simulink model "stm32f4_data_logger_ascii_rtc_demo"  (Simulink 7.3)
settings: Solver=FixedStepDiscrete  SolverMode=SingleTasking  StartTime=0.0  StopTime=10.0  RelTol=1e-3
PreLoadFcn:
  | waijung.modelPreload; % Required for working with Waijung Blockset. Do not remove.
undefined symbols (not defined in the file): HSEOSC, Link, LQFP176, ST, STM32F417IG
libraries: simulink x17, stm32f4_sdio_lib x1, stm32f4_io_lib x1, stm32f4_adc_lib x1, stm32f4_device_config_lib x1
CloseFcn:
  | waijung.modelClose; % Required for working with Waijung Blockset. Do not remove.
settings Model: Creator=Krisada  LastModifiedBy=Krisada
settings OptimizationCC: OptimizeModelRefInitCode=on  LifeSpan=1
settings HardwareCC: ProdEndianess=LittleEndian  ProdHWDeviceType=ARM Compatible->Cortex - M4  TargetEndianess=LittleEndian  TargetHWDeviceType=ARM Compatible->Cortex - M4
settings RTWCC: SystemTargetFile=stm32f4.tlc  GenerateMakefile=off  TemplateMakefile=ert_default_tmf  Description=STM32F4 Target  ProcessScript=stm32f4_make_rtw_hook
settings CodeAppCC: IgnoreCustomStorageClasses=off
settings STFCustomTargetCC: ModelReferenceCompliant=off  CombineOutputUpdateFcns=on  ERTCustomFileBanners=on  SupportContinuousTime=off  SupportNonInlinedSFcns=off  SystemTargetFile=stm32f4.tlc
settings ERTTargetCC: MultiwordLength=2048  ModelReferenceCompliant=off  ParMdlRefBuildCompliant=off  CompOptLevelCompliant=off  ERTFirstTimeCompliant=off  ModelStepFunctionPrototypeControlCompliant=off  CPPClassGenCompliant=off  ExtModeMexFile=noextcomm  InlinedParameterPlacement=NonHierarchical  ERTSrcFileBannerTemplate=stm32f4_code_template.cgt  ERTHdrFileBannerTemplate=stm32f4_code_template.cgt  ERTDataSrcFileTemplate=stm32f4_code_template.cgt  ERTDataHdrFileTemplate=stm32f4_code_template.cgt  ERTCustomFileTemplate=stm32f4_file_process.tlc

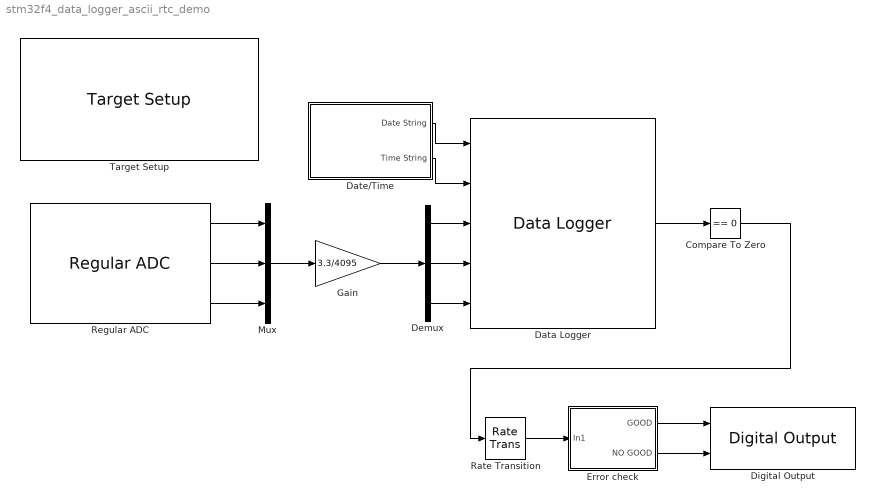
== system stm32f4_data_logger_ascii_rtc_demo ==
  Compare To Zero : simulink/Logic and Bit Operations/Compare To Zero  SystemSampleTime=-1  relop===  LogicOutDataTypeMode=uint8  ZeroCross=off
  Data Logger : stm32f4_sdio_lib/Data Logger  variablefilename=off  filename='data.csv'  conf=DataLogger  transfer=Blocking  packet=Ascii  header='Date,Time,data1,data2,data3\r\n'  asciiformat='%s,%s,%f,%f,%f,\r\n'  porttype_double=2  porttype_single=0  porttype_int8=0  porttype_uint8=1  porttype_int16=0  porttype_uint16=0  porttype_int32=0  porttype_uint32=0  advance=off  buffersize=2048  safeprintf=on  createfileoptions=Rename  synctimer=1  enablestatus=on  portpinstr=0  sampletime=-1  blockid=DataLogger  inputporttype=[-1,-1,-1,-1,-1]  inputportwidth=[1,1,1,1,1]  inputportlabel={'D0 (string)','D1 (string)','D2 (single)','D3 (single)','D4 (single)'}  outputporttype=[3]  outputportwidth=[1]  outputportlabel={'Status'}  compat=0  optionstring="[\"on\",\"off\",\"data.csv\",\"Ascii\",\"2048\",\"?\",\"?\",\"on\",\"1000000\",\"Rename\",\"-\",\"-\",\"-\",\"-\",\"-\",\"char *\",\"char *\",\"float\",\"float\",\"float\"]"
  Date/Time : Subsystem
  Demux : Demux  Outputs=3
  Digital Output : stm32f4_io_lib/Digital Output  use_bitband=on  port=D  speed=100  porttype=Push Pull  porttypestr=PP  use_pin0=off  use_pin1=off  use_pin2=off  use_pin3=off  use_pin4=off  use_pin5=off  use_pin6=off  use_pin7=off  use_pin8=off  use_pin9=off  use_pin10=off  use_pin11=off  use_pin12=on  use_pin13=on  use_pin14=off  use_pin15=off  pinstr=GPIO_Pin_12 | GPIO_Pin_13  usedpinarray="[0  0  0  0  0  0  0  0  0  0  0  0  1  1  0  0]"  bitbandingstr=|  sampletime=-1  sampletimestr=0.1  blockid=DigitalOutput  enablecustomportlabel=off  globalinit=off  cinputportlabel=In1, In2  coutputportlabel=0
      | #define DigitalOutput_D12 Peripheral_BB(GPIOD->ODR, 12)  /* Output pin */
      | #define DigitalOutput_D13 Peripheral_BB(GPIOD->ODR, 13)  /* Output pin */
  Error check : Subsystem
  Gain : Gain  Gain=3.3/4095  ParameterDataType=fixdt(1, 16)  ParameterScaling=2^0  OutDataType=fixdt(1, 16)  OutScaling=2^0  OutDataTypeStr=Inherit: Same as input  ParamDataTypeStr=Inherit: Same as input
  Mux : Mux  Inputs=3
  Rate Transition : RateTransition  OutPortSampleTime=0.1
  Regular ADC : stm32f4_adc_lib/Regular ADC  Priority=1  adcmodule=1  outputdatatype=Single  prescaler=2  prescalerstr=ADC_Prescaler_Div2  chsamplingtime=Auto  chsamplingtimestr=ADC_SampleTime_480Cycles  read_an0=off  read_an1=off  read_an2=off  read_an3=off  read_an4=off  read_an5=on  read_an6=on  read_an7=on  read_an8=off  read_an9=off  read_an10=off  read_an11=off  read_an12=off  read_an13=off  read_an14=off  read_an15=off  read_an16=off  read_an17=off  read_an18=off  pinstr=GPIO_Pin_5 | GPIO_Pin_6 | GPIO_Pin_7  usedpinarray="[0  0  0  0  0  1  1  1  0  0  0  0  0  0  0  0  0  0  0]"  usedportidarray="[0  0  0]"  usedpinidarray="[5  6  7]"  usedpinidcount=3  sampletime=0.5  blockid=RegularADC  enablecustomportlabel=off  cinputportlabel=0  coutputportlabel=Out1, Out2
  Target Setup : stm32f4_device_config_lib/Target Setup  Priority=100  compiler=GNU ARM  previous_compiler=GNU ARM  mcu=STM32F417IG (LQFP176)  mcustr=STM32F417IG  clockconfig=HSEOSC-8MHz  system_stm32f4xx_c_path=F:\trunk\targets\stm32f4_target\stm32f4\utils\system_stm32f4xx_default\STM32F40_41xxx\hseosc8mhz  showmemoryconfiguration=off  stacksize=0x2000  heapsize=0x2000  enableautocompiledownload=on  fullchiperase=off  programmerinterface=ST-Link  editctrlstr=on  compilercontrolstr=$(patsubst %, -I%, .) -mcpu=cortex-m4 -mthumb -mthumb-interwork -mfloat-abi=hard -mfpu=fpv4-sp-d16 -ffast-math -Wall -Wextra -Ofast  assemblercontrolstr=$(patsubst %, -I%, .) -mcpu=cortex-m4 -mthumb -mthumb-interwork -mfloat-abi=hard -mfpu=fpv4-sp-d16 -ffast-math -Wall -Wextra -Ofast -Wa,-amhls=$(<:.s=.lst) -D__STACK_SIZE=$(STACK_SIZE) -D__HEAP_SIZE=$(HEAP_SIZE)  linkercontrolstr=-T$(LD_SCRIPT) -g -Wl,-Map=$(MAP),--cref,--no-warn-mismatch -mcpu=cortex-m4 -mthumb -mthumb-interwork -mfloat-abi=hard -mfpu=fpv4-sp-d16 -specs=nosys.specs  runafterdownload=on  execprofile=None  profileruart=3  profilerbaud=500000  profilertxpin=D8  profilerinitstr=0.01,168000000,1680000,500000,0  manualsetsampletime=off  sampletime=0.01  blockid=TargetSetup  systickreloadvalue=1680000  hseval=8000000  lastprofileruart=3  hclk=168000000  flashorigin=0x8000000  flashlength=1024k  ramorigin=0x20000000  ramlength=128k  useextram=off
  wires:
  Data Logger/1 -> Compare To Zero/1
  Compare To Zero/1 -> Rate Transition/1
  Error check/1(GOOD) -> Digital Output/1
  Error check/2(NO GOOD) -> Digital Output/2
  Rate Transition/1 -> Error check/1(In1)
  Gain/1 -> Demux/1
  Mux/1 -> Gain/1
  Regular ADC/2 -> Mux/2
  Regular ADC/1 -> Mux/1
  Regular ADC/3 -> Mux/3
  Demux/3 -> Data Logger/5
  Demux/2 -> Data Logger/4
  Demux/1 -> Data Logger/3
  Date/Time/2(Time String) -> Data Logger/2
  Date/Time/1(Date String) -> Data Logger/1

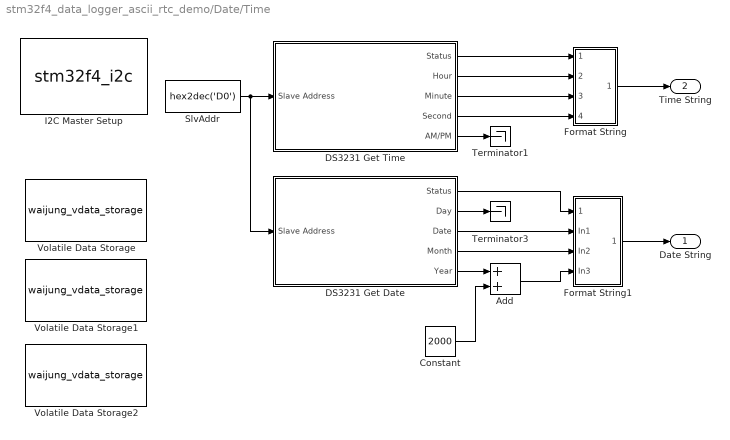
== system stm32f4_data_logger_ascii_rtc_demo/Date/Time ==
  Add : Sum  OutDataType=fixdt(1, 16)  OutScaling=2^-10
  Constant : Constant  Value=2000  OutDataTypeMode=uint32  OutDataType=fixdt(1, 16)  OutScaling=2^0  OutDataTypeStr=uint32
  DS3231 Get Date : Subsystem  mask{blockfunction=date, module=1}
      mask prompts: blockfunction "Function"; module "I2C module"
      mask init:
      | amg_high_precision_rtc_callback('init');
      mask Help: web(fullfile(waijungdocroot,'DS3231_Get_Date.htm'), '-browser')
      mask StyleString: popup(temp|time|date),popup(1|2|3)
      mask CallbackString: |amg_high_precision_rtc_callback('module');
      mask Display: text(0.5, 0.5, 'Port: I2C1','ver','middle','hor','center');port_label('input', 1,'SlvAddr');port_label('output', 1,'Status');port_label('output', 2,'Day(1-7)');port_label('output', 3,'Date(1-31)');port_label('output', 4,'Month(1-12)');port_label('output', 5,'Year(0-99)');
  DS3231 Get Time : Subsystem  mask{blockfunction=time, module=1}
      mask prompts: blockfunction "Function"; module "I2C module"
      mask init:
      | amg_high_precision_rtc_callback('init');
      mask Help: web(fullfile(waijungdocroot,'DS3231_Get_Time.htm'), '-browser')
      mask StyleString: popup(temp|time|date),popup(1|2|3)
      mask CallbackString: |amg_high_precision_rtc_callback('module');
      mask Display: text(0.5, 0.5, 'Port: I2C1','ver','middle','hor','center');port_label('input', 1,'SlvAddr');port_label('output', 1,'Status');port_label('output', 2,'Hour(0-11/23)');port_label('output', 3,'Minute(0-59)');port_label('output', 4,'Second(0-59)');port_label('output', 5,'AM(0)/PM(1)');
  Format String : Subsystem
  Format String1 : Subsystem
  I2C Master Setup : S-Function  FunctionName=stm32f4_i2c  Parameters=configuration,module,transfer,clkspeed,timeout,sdapin,sclpin,writecount,readcount,inputtypearray,outputtypearray,confstr,sampletime,sampletimestr,blockid  EnableBusSupport=off  mask(stm32f4_i2c){configuration=Setup, module=1, lastmodule=1, transfer=Blocking, dutycycle=TLow/THigh = 2, clkspeed=100, timeout=25, writecount=0, readcount=0, sdapin=B7, sclpin=B6, waitwritetime=0, inputtypearray=[0], outputtypearray=[0], confstr=["B","7","B","6","1","1","6","0","I2C_DutyCycle_2","0","off"], sampletime=-1, sampletimestr=0.01, blockid=DateTimeI2CMasterSetup}
      mask prompts: module "I2C Module"; lastmodule "Last module"; transfer "Transfer mode"; dutycycle "Duty cycle in fast mode"; clkspeed "Clock speed (kHz)"; timeout "Timeout (ms)"; writecount "Bytes write count"; readcount "Bytes read count"; sdapin "SDA pin"; sclpin "SCL pin"; waitwritetime "Wait write time (ms), default is 0"; inputtypearray "Input type array"; outputtypearray "Output type array"; confstr "Configuration string"; sampletime "Sample time (sec)"; sampletimestr "Compiled sample time (sec) in string"
      mask init:
      | stm32f4_i2c_callback('init');
      mask Help: web(fullfile(waijungdocroot,'stm32f4_i2c_setup.htm'), '-browser')
      mask StyleString: popup(Setup|Transaction),popup(1|2|3),edit,popup(Blocking|Non-blocking),popup(TLow/THigh = 16/9|TLow/THigh = 2),edit,edit,edit,edit,popup(Not used|B7|B9),popup(Not used|B6|B8),edit,edit,edit,edit,edit,edit,edit
      mask CallbackString: stm32f4_i2c_callback('configuration');|stm32f4_i2c_callback('module');|||stm32f4_i2c_callback('dutycycle');|||stm32f4_i2c_callback('writecount');|stm32f4_i2c_callback('readcount');|stm32f4_i2c_callback('sdapin');|stm32f4_i2c_callback('sclpin');||||stm32f4_i2c_callback('confstr');|stm32f4_i2c_callback('sampletime');|stm32f4_i2c_callback('sampletimestr');|stm32f4_i2c_callback('blockid');
      mask Display: text(0.5, 0.5, 'Module: I2C1\nClock: 100kHz\nSDA/SCL Pin: B7/B6','ver','middle','hor','center');
  SlvAddr : Constant  Priority=0  Value=hex2dec('D0')  OutDataTypeMode=uint8  OutDataType=fixdt(1, 16)  OutScaling=2^0  OutDataTypeStr=uint8
  Terminator1 : Terminator
  Terminator3 : Terminator
  Volatile Data Storage : S-Function  FunctionName=waijung_vdata_storage  Parameters=storagetype,storagename,initval,varname,buffersize,initvalstring,sampletime,sampletimestr,blockid,storagetypestr  EnableBusSupport=off  mask(waijung_vdata_storage){storagetype=string, storagename=date_str, initval=0, varname=DateTimeVolatileDataStorage_date_str, buffersize=64, initvalstring='', webintegration=Disable, weboutputformat='%s', webcgicallback=(void*)0, laststoragetype=string, sampletime=-1, sampletimestr=0.01, blockid=DateTimeVolatileDataStorage, storagetypestr=char}
      mask prompts: storagetype "Storage Type"; storagename "Storage Name (must be a valid variable name)"; initval "Initial value (Apply at Power on Reset only)"; varname "Variable name"; buffersize "Size (bytes)"; initvalstring "Initial value (Apply at Power on Reset only)"; webintegration "Web CGI varget/varset integration"; weboutputformat "Web CGI varget output format"; webcgicallback "Web CGI varset callback"; laststoragetype "Last selected Storage Type"; sampletime "Sample time (sec)"; sampletimestr "Compiled sample time (sec) in string"; storagetypestr "Type string"
      mask help:
      | This block implements a volatile Data Storage.
      |
      | Web CGI varset/varget integratiopn:
      | Enable - In webserver application, allow remote access via http.
      | Disable - Variable is use in local only.
      mask init:
      | waijung_vdata_storage_callback('init');
      mask Help: web(fullfile(waijungdocroot,'Volatile_Data_Storage.htm'))
      mask StyleString: popup(double|single|uint32|int32|uint16|int16|uint8|int8|string),edit,edit,edit,edit,edit,popup(Disable|ReadOnly|Write/ Read|ReadOnly with KeyValuePair|Write/ Read with KeyValuePair),edit,edit,popup(double|single|uint32|int32|uint16|int16|uint8|int8|string),edit,edit,edit,edit
      mask CallbackString: waijung_vdata_storage_callback('storagetype');|waijung_vdata_storage_callback('storagename');|waijung_vdata_storage_callback('initval');|waijung_vdata_storage_callback('varname');||waijung_vdata_storage_callback('initvalstring');|waijung_vdata_storage_callback('webintegration');|waijung_vdata_storage_callback('weboutputformat');|||waijung_vdata_storage_callback('sampletime');|waijung_vdata_storage_callback('sampletimestr');|waijung_vdata_storage_callback('blockid');|
      mask Display: text(0.5, 0.5, 'Name: date_str\nType: string','ver','middle','hor','center')
  Volatile Data Storage1 : S-Function  FunctionName=waijung_vdata_storage  Parameters=storagetype,storagename,initval,varname,buffersize,initvalstring,sampletime,sampletimestr,blockid,storagetypestr  EnableBusSupport=off  mask(waijung_vdata_storage){storagetype=string, storagename=time_str, initval=0, varname=DateTimeVolatileDataStorage1_time_str, buffersize=64, initvalstring='', webintegration=Disable, weboutputformat='%s', webcgicallback=(void*)0, laststoragetype=string, sampletime=-1, sampletimestr=0.01, blockid=DateTimeVolatileDataStorage1, storagetypestr=char}
      mask prompts: storagetype "Storage Type"; storagename "Storage Name (must be a valid variable name)"; initval "Initial value (Apply at Power on Reset only)"; varname "Variable name"; buffersize "Size (bytes)"; initvalstring "Initial value (Apply at Power on Reset only)"; webintegration "Web CGI varget/varset integration"; weboutputformat "Web CGI varget output format"; webcgicallback "Web CGI varset callback"; laststoragetype "Last selected Storage Type"; sampletime "Sample time (sec)"; sampletimestr "Compiled sample time (sec) in string"; storagetypestr "Type string"
      mask help:
      | This block implements a volatile Data Storage.
      |
      | Web CGI varset/varget integratiopn:
      | Enable - In webserver application, allow remote access via http.
      | Disable - Variable is use in local only.
      mask init:
      | waijung_vdata_storage_callback('init');
      mask Help: web(fullfile(waijungdocroot,'Volatile_Data_Storage.htm'))
      mask StyleString: popup(double|single|uint32|int32|uint16|int16|uint8|int8|string),edit,edit,edit,edit,edit,popup(Disable|ReadOnly|Write/ Read|ReadOnly with KeyValuePair|Write/ Read with KeyValuePair),edit,edit,popup(double|single|uint32|int32|uint16|int16|uint8|int8|string),edit,edit,edit,edit
      mask CallbackString: waijung_vdata_storage_callback('storagetype');|waijung_vdata_storage_callback('storagename');|waijung_vdata_storage_callback('initval');|waijung_vdata_storage_callback('varname');||waijung_vdata_storage_callback('initvalstring');|waijung_vdata_storage_callback('webintegration');|waijung_vdata_storage_callback('weboutputformat');|||waijung_vdata_storage_callback('sampletime');|waijung_vdata_storage_callback('sampletimestr');|waijung_vdata_storage_callback('blockid');|
      mask Display: text(0.5, 0.5, 'Name: time_str\nType: string','ver','middle','hor','center')
  Volatile Data Storage2 : S-Function  FunctionName=waijung_vdata_storage  Parameters=storagetype,storagename,initval,varname,buffersize,initvalstring,sampletime,sampletimestr,blockid,storagetypestr  EnableBusSupport=off  mask(waijung_vdata_storage){storagetype=string, storagename=date_time_error, initval=0, varname=DateTimeVolatileDataStorage2_date_time_error, buffersize=64, initvalstring='Error', webintegration=Disable, weboutputformat='%s', webcgicallback=(void*)0, laststoragetype=string, sampletime=-1, sampletimestr=0.01, blockid=DateTimeVolatileDataStorage2, storagetypestr=char}
      mask prompts: storagetype "Storage Type"; storagename "Storage Name (must be a valid variable name)"; initval "Initial value (Apply at Power on Reset only)"; varname "Variable name"; buffersize "Size (bytes)"; initvalstring "Initial value (Apply at Power on Reset only)"; webintegration "Web CGI varget/varset integration"; weboutputformat "Web CGI varget output format"; webcgicallback "Web CGI varset callback"; laststoragetype "Last selected Storage Type"; sampletime "Sample time (sec)"; sampletimestr "Compiled sample time (sec) in string"; storagetypestr "Type string"
      mask help:
      | This block implements a volatile Data Storage.
      |
      | Web CGI varset/varget integratiopn:
      | Enable - In webserver application, allow remote access via http.
      | Disable - Variable is use in local only.
      mask init:
      | waijung_vdata_storage_callback('init');
      mask Help: web(fullfile(waijungdocroot,'Volatile_Data_Storage.htm'))
      mask StyleString: popup(double|single|uint32|int32|uint16|int16|uint8|int8|string),edit,edit,edit,edit,edit,popup(Disable|ReadOnly|Write/ Read|ReadOnly with KeyValuePair|Write/ Read with KeyValuePair),edit,edit,popup(double|single|uint32|int32|uint16|int16|uint8|int8|string),edit,edit,edit,edit
      mask CallbackString: waijung_vdata_storage_callback('storagetype');|waijung_vdata_storage_callback('storagename');|waijung_vdata_storage_callback('initval');|waijung_vdata_storage_callback('varname');||waijung_vdata_storage_callback('initvalstring');|waijung_vdata_storage_callback('webintegration');|waijung_vdata_storage_callback('weboutputformat');|||waijung_vdata_storage_callback('sampletime');|waijung_vdata_storage_callback('sampletimestr');|waijung_vdata_storage_callback('blockid');|
      mask Display: text(0.5, 0.5, 'Name: date_time_error\nType: string','ver','middle','hor','center')
  Date String : Outport  OutDataType=fixdt(1, 16)  OutScaling=2^0
  Time String : Outport  Port=2  OutDataType=fixdt(1, 16)  OutScaling=2^0
  wires:
  SlvAddr/1 -> DS3231 Get Time/1(Slave Address), DS3231 Get Date/1(Slave Address)
  DS3231 Get Time/1(Status) -> Format String/1(Status)
  DS3231 Get Time/5(AM/PM) -> Terminator1/1
  DS3231 Get Date/1(Status) -> Format String1/1(Status)
  DS3231 Get Date/2(Day) -> Terminator3/1
  DS3231 Get Time/2(Hour) -> Format String/2(In1)
  DS3231 Get Date/3(Date) -> Format String1/2(In1)
  DS3231 Get Date/4(Month) -> Format String1/3(In2)
  Add/1 -> Format String1/4(In3)
  DS3231 Get Date/5(Year) -> Add/1
  Constant/1 -> Add/2
  DS3231 Get Time/3(Minute) -> Format String/3(In2)
  DS3231 Get Time/4(Second) -> Format String/4(In3)
  Format String/1(Time) -> Time String/1
  Format String1/1(Date) -> Date String/1

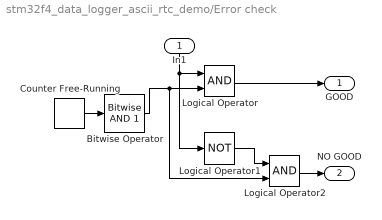
== system stm32f4_data_logger_ascii_rtc_demo/Error check ==
  In1 : Inport
  Bitwise Operator : simulink/Logic and Bit Operations/Bitwise Operator  logicop=AND  UseBitMask=on  BitMask=1  BitMaskRealWorld=Stored Integer
  Counter Free-Running : simulink/Sources/Counter Free-Running  SystemSampleTime=-1  NumBits=16  tsamp=-1
  Logical Operator : Logic  AllPortsSameDT=off  OutDataTypeMode=boolean  LogicDataType=fixdt(0, 8)  OutDataTypeStr=boolean
  Logical Operator1 : Logic  Operator=NOT  AllPortsSameDT=off  OutDataTypeMode=boolean  LogicDataType=fixdt(0, 8)  OutDataTypeStr=boolean
  Logical Operator2 : Logic  AllPortsSameDT=off  OutDataTypeMode=boolean  LogicDataType=fixdt(0, 8)  OutDataTypeStr=boolean
  GOOD : Outport
  NO GOOD : Outport  Port=2
  wires:
  In1/1 -> Logical Operator1/1, Logical Operator/1
  Bitwise Operator/1 -> Logical Operator/2, Logical Operator2/2
  Logical Operator1/1 -> Logical Operator2/1
  Counter Free-Running/1 -> Bitwise Operator/1
  Logical Operator/1 -> GOOD/1
  Logical Operator2/1 -> NO GOOD/1

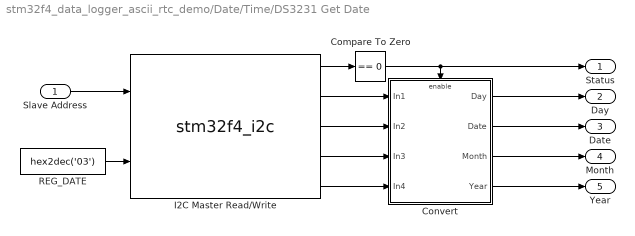
== system stm32f4_data_logger_ascii_rtc_demo/Date/Time/DS3231 Get Date ==
  Slave Address : Inport  OutDataType=fixdt(1, 16)  OutScaling=2^0
  Compare To Zero : simulink/Logic and Bit Operations/Compare To Zero  SystemSampleTime=-1  relop===  LogicOutDataTypeMode=uint8  ZeroCross=off
  Convert : Subsystem  TreatAsAtomicUnit=on
  I2C Master Read/Write : S-Function  FunctionName=stm32f4_i2c  Parameters=configuration,module,transfer,clkspeed,timeout,sdapin,sclpin,writecount,readcount,inputtypearray,outputtypearray,confstr,sampletime,sampletimestr,blockid  EnableBusSupport=off  mask(stm32f4_i2c){configuration=Transaction, module=1, lastmodule=3, transfer=Blocking, dutycycle=TLow/THigh = 2, clkspeed=400, timeout=25, writecount=1, readcount=4, sdapin=C9, sclpin=A8, waitwritetime=0, inputtypearray=[2 3 3], outputtypearray=[5 3 3 3 3 3], confstr=["C","9","A","8","1","1","6","0","I2C_DutyCycle_2","0","off"], sampletime=-1, sampletimestr=0.5, blockid=DateTimeDS3231GetDateI2CMasterReadWrite}
      mask prompts: module "I2C Module"; lastmodule "Last module"; transfer "Transfer mode"; dutycycle "Duty cycle in fast mode"; clkspeed "Clock speed (kHz)"; timeout "Timeout (ms)"; writecount "Bytes write count"; readcount "Bytes read count"; sdapin "SDA pin"; sclpin "SCL pin"; waitwritetime "Wait write time (ms), default is 0"; inputtypearray "Input type array"; outputtypearray "Output type array"; confstr "Configuration string"; sampletime "Sample time (sec)"; sampletimestr "Compiled sample time (sec) in string"
      mask init:
      | stm32f4_i2c_callback('init');
      mask Help: web(fullfile(waijungdocroot,'stm32f4_i2c_readwrite.htm'), '-browser')
      mask StyleString: popup(Setup|Transaction),popup(1|2|3),edit,popup(Blocking|Non-blocking),popup(TLow/THigh = 16/9|TLow/THigh = 2),edit,edit,edit,edit,popup(-|C9),popup(-|A8),edit,edit,edit,edit,edit,edit,edit
      mask CallbackString: stm32f4_i2c_callback('configuration');|stm32f4_i2c_callback('module');|||stm32f4_i2c_callback('dutycycle');|||stm32f4_i2c_callback('writecount');|stm32f4_i2c_callback('readcount');|stm32f4_i2c_callback('sdapin');|stm32f4_i2c_callback('sclpin');||||stm32f4_i2c_callback('confstr');|stm32f4_i2c_callback('sampletime');|stm32f4_i2c_callback('sampletimestr');|stm32f4_i2c_callback('blockid');
      mask Display: text(0.5, 0.5, 'Module: I2C1\nTransfer: Blocking\nWrite: 1 bytes\nRead: 4 bytes\nTs (sec): 0.5','ver','middle','hor','center');port_label('input', 1,'SlvAddr');port_label('input', 2,'Wr0 (uint8)');port_label('output', 1,'Status');port_label('output', 2,'Rd0 (uint8)');port_label('output', 3,'Rd1 (uint8)');port_label('output', 4,'Rd2 (uint8)');port_label('output', 5,'Rd3 (uint8)');
  REG_DATE : Constant  Value=hex2dec('03')  OutDataTypeMode=uint8  OutDataType=fixdt(1, 16)  OutScaling=2^0  OutDataTypeStr=uint8
  Status : Outport
  Day : Outport  Port=2
  Date : Outport  Port=3
  Month : Outport  Port=4
  Year : Outport  Port=5
  wires:
  Convert/3(Month) -> Month/1
  Convert/4(Year) -> Year/1
  Convert/2(Date) -> Date/1
  Convert/1(Day) -> Day/1
  I2C Master Read/Write/5 -> Convert/4(In4)
  REG_DATE/1 -> I2C Master Read/Write/2
  Slave Address/1 -> I2C Master Read/Write/1
  I2C Master Read/Write/1 -> Compare To Zero/1
  Compare To Zero/1 -> Convert/Enable, Status/1
  I2C Master Read/Write/2 -> Convert/1(In1)
  I2C Master Read/Write/3 -> Convert/2(In2)
  I2C Master Read/Write/4 -> Convert/3(In3)

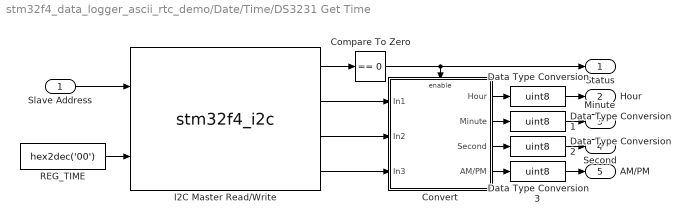
== system stm32f4_data_logger_ascii_rtc_demo/Date/Time/DS3231 Get Time ==
  Slave Address : Inport  OutDataType=fixdt(1, 16)  OutScaling=2^0
  Compare To Zero : simulink/Logic and Bit Operations/Compare To Zero  SystemSampleTime=-1  relop===  LogicOutDataTypeMode=uint8  ZeroCross=off
  Convert : Subsystem  TreatAsAtomicUnit=on
  Data Type Conversion{,1..3} (4 alike) : DataTypeConversion  OutDataTypeMode=uint8  OutDataType=fixdt(1, 16)  OutScaling=2^0  OutDataTypeStr=uint8
  I2C Master Read/Write : S-Function  FunctionName=stm32f4_i2c  Parameters=configuration,module,transfer,clkspeed,timeout,sdapin,sclpin,writecount,readcount,inputtypearray,outputtypearray,confstr,sampletime,sampletimestr,blockid  EnableBusSupport=off  mask(stm32f4_i2c){configuration=Transaction, module=1, lastmodule=3, transfer=Blocking, dutycycle=TLow/THigh = 2, clkspeed=400, timeout=25, writecount=1, readcount=3, sdapin=C9, sclpin=A8, waitwritetime=0, inputtypearray=[2 3 3], outputtypearray=[4 3 3 3 3], confstr=["C","9","A","8","1","1","6","0","I2C_DutyCycle_2","0","off"], sampletime=-1, sampletimestr=0.5, blockid=DateTimeDS3231GetTimeI2CMasterReadWrite}
      mask prompts: module "I2C Module"; lastmodule "Last module"; transfer "Transfer mode"; dutycycle "Duty cycle in fast mode"; clkspeed "Clock speed (kHz)"; timeout "Timeout (ms)"; writecount "Bytes write count"; readcount "Bytes read count"; sdapin "SDA pin"; sclpin "SCL pin"; waitwritetime "Wait write time (ms), default is 0"; inputtypearray "Input type array"; outputtypearray "Output type array"; confstr "Configuration string"; sampletime "Sample time (sec)"; sampletimestr "Compiled sample time (sec) in string"
      mask init:
      | stm32f4_i2c_callback('init');
      mask Help: web(fullfile(waijungdocroot,'stm32f4_i2c_readwrite.htm'), '-browser')
      mask StyleString: popup(Setup|Transaction),popup(1|2|3),edit,popup(Blocking|Non-blocking),popup(TLow/THigh = 16/9|TLow/THigh = 2),edit,edit,edit,edit,popup(-|C9),popup(-|A8),edit,edit,edit,edit,edit,edit,edit
      mask CallbackString: stm32f4_i2c_callback('configuration');|stm32f4_i2c_callback('module');|||stm32f4_i2c_callback('dutycycle');|||stm32f4_i2c_callback('writecount');|stm32f4_i2c_callback('readcount');|stm32f4_i2c_callback('sdapin');|stm32f4_i2c_callback('sclpin');||||stm32f4_i2c_callback('confstr');|stm32f4_i2c_callback('sampletime');|stm32f4_i2c_callback('sampletimestr');|stm32f4_i2c_callback('blockid');
      mask Display: text(0.5, 0.5, 'Module: I2C1\nTransfer: Blocking\nWrite: 1 bytes\nRead: 3 bytes\nTs (sec): 0.5','ver','middle','hor','center');port_label('input', 1,'SlvAddr');port_label('input', 2,'Wr0 (uint8)');port_label('output', 1,'Status');port_label('output', 2,'Rd0 (uint8)');port_label('output', 3,'Rd1 (uint8)');port_label('output', 4,'Rd2 (uint8)');
  REG_TIME : Constant  Value=hex2dec('00')  OutDataTypeMode=uint8  OutDataType=fixdt(1, 16)  OutScaling=2^0  OutDataTypeStr=uint8
  Status : Outport
  Hour : Outport  Port=2
  Minute : Outport  Port=3
  Second : Outport  Port=4
  AM/PM : Outport  Port=5
  wires:
  Data Type Conversion3/1 -> AM/PM/1
  Data Type Conversion2/1 -> Second/1
  Data Type Conversion1/1 -> Minute/1
  Data Type Conversion/1 -> Hour/1
  Convert/4(AM/PM) -> Data Type Conversion3/1
  Convert/1(Hour) -> Data Type Conversion/1
  Convert/2(Minute) -> Data Type Conversion1/1
  Convert/3(Second) -> Data Type Conversion2/1
  I2C Master Read/Write/4 -> Convert/3(In3)
  I2C Master Read/Write/3 -> Convert/2(In2)
  I2C Master Read/Write/2 -> Convert/1(In1)
  Compare To Zero/1 -> Status/1, Convert/Enable
  I2C Master Read/Write/1 -> Compare To Zero/1
  Slave Address/1 -> I2C Master Read/Write/1
  REG_TIME/1 -> I2C Master Read/Write/2

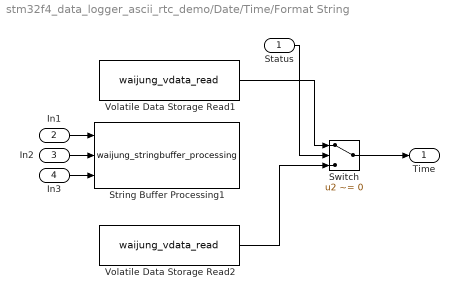
== system stm32f4_data_logger_ascii_rtc_demo/Date/Time/Format String ==
  Status : Inport
  In1 : Inport  Port=2
  In2 : Inport  Port=3
  In3 : Inport  Port=4
  String Buffer Processing1 : S-Function  FunctionName=waijung_stringbuffer_processing  Parameters=configuration,varname,sformat,porttypes,portcount,inputtypearray,outputtypearray,sampletime,sampletimestr,blockid  EnableBusSupport=off  mask(waijung_stringbuffer_processing){configuration=sprintf, storagename=time_str, sformat='%2u:%2u:%2u', enableoutput=off, varname=DateTimeVolatileDataStorage1_time_str, inputtypearray=[3 -1 -1 -1], outputtypearray=[0], porttypes=["uint32_t","uint32_t","uint32_t"], portcount=3, sampletime=-1, sampletimestr=0.5, blockid=DateTimeFormatStringStringBufferProcessing1}
      mask prompts: configuration "Function"; storagename "String buffer"; sformat "Printf format"; enableoutput "Enable output status"; varname "Variable name"; inputtypearray "Input type array"; outputtypearray "Output type array"; porttypes "Port type list"; portcount "Port type count"; sampletime "Sample time (sec)"; sampletimestr "Compiled sample time (sec) in string"
      mask help:
      | This block implements string processing, sprintf/ sscanf command.
      | Supported format:
      | %u, %i, %o, %x: uint32
      | %d: int32
      | %e, %g, %f: single
      | %c: int8
      |
      | Status:
      |  0: Failed.
      |  Non-zero: Success.
      mask init:
      | waijung_stringbuffer_processing_callback('init');
      mask Help: web(fullfile(waijungdocroot,'String_Buffer_Processing.htm'))
      mask StyleString: popup(sprintf|sscanf),popup(date_str|time_str|date_time_error|<output>),edit,checkbox,edit,edit,edit,edit,edit,edit,edit,edit
      mask CallbackString: waijung_stringbuffer_processing_callback('configuration');||waijung_stringbuffer_processing_callback('sformat');|waijung_stringbuffer_processing_callback('enableoutput');||||||waijung_stringbuffer_processing_callback('sampletime');|waijung_stringbuffer_processing_callback('sampletimestr');|waijung_stringbuffer_processing_callback('blockid');
      mask Display: text(0.5, 0.5, '[ sprintf ]\nBuffer: time_str\nTs (sec): 0.5','ver','middle','hor','center');port_label('input', 1,'%u');port_label('input', 2,'%u');port_label('input', 3,'%u');
  Switch : Switch  Criteria=u2 ~= 0  OutDataType=fixdt(1, 16)  OutScaling=2^0
  Volatile Data Storage Read1 : S-Function  FunctionName=waijung_vdata_read  Parameters=storagename,varname,sampletime,sampletimestr,blockid,storagetype,storagetypestr  EnableBusSupport=off  mask(waijung_vdata_read){storagename=time_str, varname=DateTimeVolatileDataStorage1_time_str, sampletime=inf, sampletimestr=0.5, blockid=DateTimeFormatStringVolatileDataStorageRead1, storagetype=string, storagetypestr=uint32_t}
      mask prompts: storagename "Storage Name"; varname "Variable name"; sampletime "Sample time (sec)"; sampletimestr "Compiled sample time (sec) in string"; storagetype "Data type"; storagetypestr "Data type string"
      mask help: This block implements read data from a buffer.
      mask init:
      | waijung_vdata_read_callback('init');
      mask Help: web(fullfile(waijungdocroot,'Volatile_Data_Storage_Read.htm'))
      mask StyleString: popup(date_str|time_str|date_time_error),edit,edit,edit,edit,edit,edit
      mask CallbackString: waijung_vdata_read_callback('storagename');|waijung_vdata_read_callback('varname');|waijung_vdata_read_callback('sampletime');|waijung_vdata_read_callback('sampletimestr');|waijung_vdata_read_callback('blockid');|waijung_vdata_read_callback('storagetype');|
      mask Display: text(0.05, 0.5, 'Buffer: time_str','ver','middle','hor','left');port_label('output',1,'D1(string)')
  Volatile Data Storage Read2 : S-Function  FunctionName=waijung_vdata_read  Parameters=storagename,varname,sampletime,sampletimestr,blockid,storagetype,storagetypestr  EnableBusSupport=off  mask(waijung_vdata_read){storagename=date_time_error, varname=DateTimeVolatileDataStorage2_date_time_error, sampletime=inf, sampletimestr=0.5, blockid=DateTimeFormatStringVolatileDataStorageRead2, storagetype=string, storagetypestr=uint32_t}
      mask prompts: storagename "Storage Name"; varname "Variable name"; sampletime "Sample time (sec)"; sampletimestr "Compiled sample time (sec) in string"; storagetype "Data type"; storagetypestr "Data type string"
      mask help: This block implements read data from a buffer.
      mask init:
      | waijung_vdata_read_callback('init');
      mask Help: web(fullfile(waijungdocroot,'Volatile_Data_Storage_Read.htm'))
      mask StyleString: popup(date_str|time_str|date_time_error),edit,edit,edit,edit,edit,edit
      mask CallbackString: waijung_vdata_read_callback('storagename');|waijung_vdata_read_callback('varname');|waijung_vdata_read_callback('sampletime');|waijung_vdata_read_callback('sampletimestr');|waijung_vdata_read_callback('blockid');|waijung_vdata_read_callback('storagetype');|
      mask Display: text(0.05, 0.5, 'Buffer: date_time_error','ver','middle','hor','left');port_label('output',1,'D1(string)')
  Time : Outport
  wires:
  In1/1 -> String Buffer Processing1/1
  In2/1 -> String Buffer Processing1/2
  Switch/1 -> Time/1
  In3/1 -> String Buffer Processing1/3
  Status/1 -> Switch/2
  Volatile Data Storage Read2/1 -> Switch/3
  Volatile Data Storage Read1/1 -> Switch/1

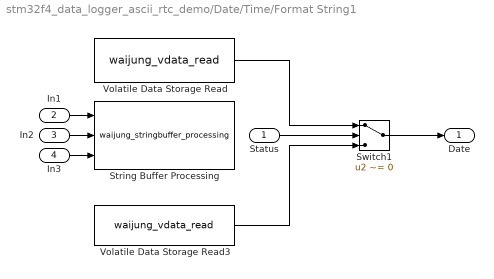
== system stm32f4_data_logger_ascii_rtc_demo/Date/Time/Format String1 ==
  Status : Inport
  In1 : Inport  Port=2
  In2 : Inport  Port=3
  In3 : Inport  Port=4
  String Buffer Processing : S-Function  FunctionName=waijung_stringbuffer_processing  Parameters=configuration,varname,sformat,porttypes,portcount,inputtypearray,outputtypearray,sampletime,sampletimestr,blockid  EnableBusSupport=off  mask(waijung_stringbuffer_processing){configuration=sprintf, storagename=date_str, sformat='%2u/%2u/%2u', enableoutput=off, varname=DateTimeVolatileDataStorage_date_str, inputtypearray=[3 -1 -1 -1], outputtypearray=[0], porttypes=["uint32_t","uint32_t","uint32_t"], portcount=3, sampletime=-1, sampletimestr=0.5, blockid=DateTimeFormatString1StringBufferProcessing}
      mask prompts: configuration "Function"; storagename "String buffer"; sformat "Printf format"; enableoutput "Enable output status"; varname "Variable name"; inputtypearray "Input type array"; outputtypearray "Output type array"; porttypes "Port type list"; portcount "Port type count"; sampletime "Sample time (sec)"; sampletimestr "Compiled sample time (sec) in string"
      mask help:
      | This block implements string processing, sprintf/ sscanf command.
      | Supported format:
      | %u, %i, %o, %x: uint32
      | %d: int32
      | %e, %g, %f: single
      | %c: int8
      |
      | Status:
      |  0: Failed.
      |  Non-zero: Success.
      mask init:
      | waijung_stringbuffer_processing_callback('init');
      mask Help: web(fullfile(waijungdocroot,'String_Buffer_Processing.htm'))
      mask StyleString: popup(sprintf|sscanf),popup(date_str|time_str|date_time_error|<output>),edit,checkbox,edit,edit,edit,edit,edit,edit,edit,edit
      mask CallbackString: waijung_stringbuffer_processing_callback('configuration');||waijung_stringbuffer_processing_callback('sformat');|waijung_stringbuffer_processing_callback('enableoutput');||||||waijung_stringbuffer_processing_callback('sampletime');|waijung_stringbuffer_processing_callback('sampletimestr');|waijung_stringbuffer_processing_callback('blockid');
      mask Display: text(0.5, 0.5, '[ sprintf ]\nBuffer: date_str\nTs (sec): 0.5','ver','middle','hor','center');port_label('input', 1,'%u');port_label('input', 2,'%u');port_label('input', 3,'%u');
  Switch1 : Switch  Criteria=u2 ~= 0  OutDataType=fixdt(1, 16)  OutScaling=2^0
  Volatile Data Storage Read : S-Function  FunctionName=waijung_vdata_read  Parameters=storagename,varname,sampletime,sampletimestr,blockid,storagetype,storagetypestr  EnableBusSupport=off  mask(waijung_vdata_read){storagename=date_str, varname=DateTimeVolatileDataStorage_date_str, sampletime=inf, sampletimestr=0.5, blockid=DateTimeFormatString1VolatileDataStorageRead, storagetype=string, storagetypestr=uint32_t}
      mask prompts: storagename "Storage Name"; varname "Variable name"; sampletime "Sample time (sec)"; sampletimestr "Compiled sample time (sec) in string"; storagetype "Data type"; storagetypestr "Data type string"
      mask help: This block implements read data from a buffer.
      mask init:
      | waijung_vdata_read_callback('init');
      mask Help: web(fullfile(waijungdocroot,'Volatile_Data_Storage_Read.htm'))
      mask StyleString: popup(date_str|time_str|date_time_error),edit,edit,edit,edit,edit,edit
      mask CallbackString: waijung_vdata_read_callback('storagename');|waijung_vdata_read_callback('varname');|waijung_vdata_read_callback('sampletime');|waijung_vdata_read_callback('sampletimestr');|waijung_vdata_read_callback('blockid');|waijung_vdata_read_callback('storagetype');|
      mask Display: text(0.05, 0.5, 'Buffer: date_str','ver','middle','hor','left');port_label('output',1,'D1(string)')
  Volatile Data Storage Read3 : S-Function  FunctionName=waijung_vdata_read  Parameters=storagename,varname,sampletime,sampletimestr,blockid,storagetype,storagetypestr  EnableBusSupport=off  mask(waijung_vdata_read){storagename=date_time_error, varname=DateTimeVolatileDataStorage2_date_time_error, sampletime=inf, sampletimestr=0.5, blockid=DateTimeFormatString1VolatileDataStorageRead3, storagetype=string, storagetypestr=uint32_t}
      mask prompts: storagename "Storage Name"; varname "Variable name"; sampletime "Sample time (sec)"; sampletimestr "Compiled sample time (sec) in string"; storagetype "Data type"; storagetypestr "Data type string"
      mask help: This block implements read data from a buffer.
      mask init:
      | waijung_vdata_read_callback('init');
      mask Help: web(fullfile(waijungdocroot,'Volatile_Data_Storage_Read.htm'))
      mask StyleString: popup(date_str|time_str|date_time_error),edit,edit,edit,edit,edit,edit
      mask CallbackString: waijung_vdata_read_callback('storagename');|waijung_vdata_read_callback('varname');|waijung_vdata_read_callback('sampletime');|waijung_vdata_read_callback('sampletimestr');|waijung_vdata_read_callback('blockid');|waijung_vdata_read_callback('storagetype');|
      mask Display: text(0.05, 0.5, 'Buffer: date_time_error','ver','middle','hor','left');port_label('output',1,'D1(string)')
  Date : Outport
  wires:
  In1/1 -> String Buffer Processing/1
  In2/1 -> String Buffer Processing/2
  Switch1/1 -> Date/1
  In3/1 -> String Buffer Processing/3
  Status/1 -> Switch1/2
  Volatile Data Storage Read3/1 -> Switch1/3
  Volatile Data Storage Read/1 -> Switch1/1

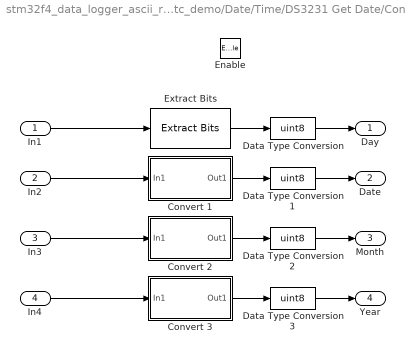
== system stm32f4_data_logger_ascii_rtc_demo/Date/Time/DS3231 Get Date/Convert ==
  In1 : Inport  OutDataType=fixdt(1, 16)  OutScaling=2^0
  In2 : Inport  Port=2  OutDataType=fixdt(1, 16)  OutScaling=2^0
  In3 : Inport  Port=3  OutDataType=fixdt(1, 16)  OutScaling=2^0
  In4 : Inport  Port=4  OutDataType=fixdt(1, 16)  OutScaling=2^0
  Enable : EnablePort
  Convert 1 : Subsystem
  Convert 2 : Subsystem
  Convert 3 : Subsystem
  Data Type Conversion{,1..3} (4 alike) : DataTypeConversion  OutDataTypeMode=uint8  OutDataType=fixdt(1, 16)  OutScaling=2^0  OutDataTypeStr=uint8
  Extract Bits : simulink/Logic and Bit Operations/Extract Bits  SystemSampleTime=-1  bitsToExtract=Range of bits  numBits=8  bitIdxRange=[0 3]  outScalingMode=Treat bit field as an integer
  Day : Outport  OutDataType=fixdt(1, 16)  OutScaling=2^0
  Date : Outport  Port=2  OutDataType=fixdt(1, 16)  OutScaling=2^0
  Month : Outport  Port=3  OutDataType=fixdt(1, 16)  OutScaling=2^0
  Year : Outport  Port=4  OutDataType=fixdt(1, 16)  OutScaling=2^0
  wires:
  Data Type Conversion3/1 -> Year/1
  Data Type Conversion2/1 -> Month/1
  Data Type Conversion1/1 -> Date/1
  Data Type Conversion/1 -> Day/1
  Convert 3/1(Out1) -> Data Type Conversion3/1
  In4/1 -> Convert 3/1(In1)
  Convert 2/1(Out1) -> Data Type Conversion2/1
  In3/1 -> Convert 2/1(In1)
  In2/1 -> Convert 1/1(In1)
  Convert 1/1(Out1) -> Data Type Conversion1/1
  Extract Bits/1 -> Data Type Conversion/1
  In1/1 -> Extract Bits/1

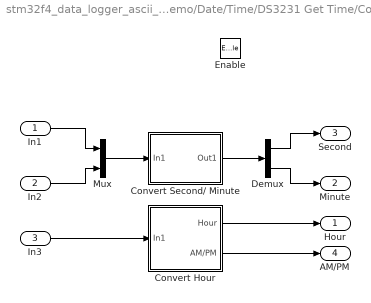
== system stm32f4_data_logger_ascii_rtc_demo/Date/Time/DS3231 Get Time/Convert ==
  In1 : Inport  OutDataType=fixdt(1, 16)  OutScaling=2^0
  In2 : Inport  Port=2  OutDataType=fixdt(1, 16)  OutScaling=2^0
  In3 : Inport  Port=3  OutDataType=fixdt(1, 16)  OutScaling=2^0
  Enable : EnablePort
  Convert Hour : Subsystem
  Convert Second/ Minute : Subsystem
  Demux : Demux  Outputs=2
  Mux : Mux  Inputs=2
  Hour : Outport  OutDataType=fixdt(1, 16)  OutScaling=2^0
  Minute : Outport  Port=2  OutDataType=fixdt(1, 16)  OutScaling=2^0
  Second : Outport  Port=3  OutDataType=fixdt(1, 16)  OutScaling=2^0
  AM/PM : Outport  Port=4  OutDataType=fixdt(1, 16)  OutScaling=2^0
  wires:
  Convert Hour/2(AM/PM) -> AM/PM/1
  Convert Hour/1(Hour) -> Hour/1
  In3/1 -> Convert Hour/1(In1)
  Demux/2 -> Minute/1
  Demux/1 -> Second/1
  Convert Second/ Minute/1(Out1) -> Demux/1
  Mux/1 -> Convert Second/ Minute/1(In1)
  In1/1 -> Mux/1
  In2/1 -> Mux/2

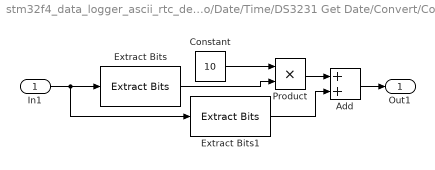
== system stm32f4_data_logger_ascii_rtc_demo/Date/Time/DS3231 Get Date/Convert/Convert 1 ==
  In1 : Inport
  Add : Sum  OutDataType=fixdt(1, 16)  OutScaling=2^-10
  Constant : Constant  Value=10  OutDataTypeMode=uint8  OutDataType=fixdt(1, 16)  OutScaling=2^0  OutDataTypeStr=uint8
  Extract Bits : simulink/Logic and Bit Operations/Extract Bits  SystemSampleTime=-1  bitsToExtract=Range of bits  numBits=8  bitIdxRange=[4 5]  outScalingMode=Treat bit field as an integer
  Extract Bits1 : simulink/Logic and Bit Operations/Extract Bits  SystemSampleTime=-1  bitsToExtract=Range of bits  numBits=8  bitIdxRange=[0 3]  outScalingMode=Treat bit field as an integer
  Product : Product  OutDataType=fixdt(1, 16)  OutScaling=2^0  RndMeth=Zero
  Out1 : Outport
  wires:
  Add/1 -> Out1/1
  Extract Bits1/1 -> Add/2
  Product/1 -> Add/1
  Extract Bits/1 -> Product/2
  Constant/1 -> Product/1
  In1/1 -> Extract Bits1/1, Extract Bits/1

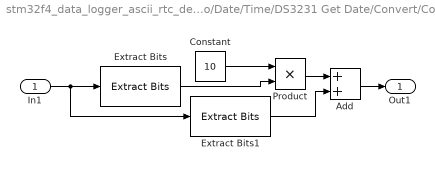
== system stm32f4_data_logger_ascii_rtc_demo/Date/Time/DS3231 Get Date/Convert/Convert 2 ==
  In1 : Inport
  Add : Sum  OutDataType=fixdt(1, 16)  OutScaling=2^-10
  Constant : Constant  Value=10  OutDataTypeMode=uint8  OutDataType=fixdt(1, 16)  OutScaling=2^0  OutDataTypeStr=uint8
  Extract Bits : simulink/Logic and Bit Operations/Extract Bits  SystemSampleTime=-1  bitsToExtract=Range of bits  numBits=8  bitIdxRange=[4 4]  outScalingMode=Treat bit field as an integer
  Extract Bits1 : simulink/Logic and Bit Operations/Extract Bits  SystemSampleTime=-1  bitsToExtract=Range of bits  numBits=8  bitIdxRange=[0 3]  outScalingMode=Treat bit field as an integer
  Product : Product  OutDataType=fixdt(1, 16)  OutScaling=2^0  RndMeth=Zero
  Out1 : Outport
  wires:
  In1/1 -> Extract Bits/1, Extract Bits1/1
  Constant/1 -> Product/1
  Extract Bits/1 -> Product/2
  Product/1 -> Add/1
  Extract Bits1/1 -> Add/2
  Add/1 -> Out1/1

== system stm32f4_data_logger_ascii_rtc_demo/Date/Time/DS3231 Get Date/Convert/Convert 3 ==
  In1 : Inport
  Add : Sum  OutDataType=fixdt(1, 16)  OutScaling=2^-10
  Constant : Constant  Value=10  OutDataTypeMode=uint8  OutDataType=fixdt(1, 16)  OutScaling=2^0  OutDataTypeStr=uint8
  Extract Bits : simulink/Logic and Bit Operations/Extract Bits  SystemSampleTime=-1  bitsToExtract=Range of bits  numBits=8  bitIdxRange=[4 7]  outScalingMode=Treat bit field as an integer
  Extract Bits1 : simulink/Logic and Bit Operations/Extract Bits  SystemSampleTime=-1  bitsToExtract=Range of bits  numBits=8  bitIdxRange=[0 3]  outScalingMode=Treat bit field as an integer
  Product : Product  OutDataType=fixdt(1, 16)  OutScaling=2^0  RndMeth=Zero
  Out1 : Outport
  wires:
  Add/1 -> Out1/1
  Extract Bits1/1 -> Add/2
  Product/1 -> Add/1
  Extract Bits/1 -> Product/2
  Constant/1 -> Product/1
  In1/1 -> Extract Bits1/1, Extract Bits/1

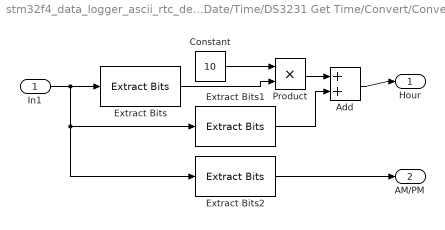
== system stm32f4_data_logger_ascii_rtc_demo/Date/Time/DS3231 Get Time/Convert/Convert Hour ==
  In1 : Inport
  Add : Sum  OutDataType=fixdt(1, 16)  OutScaling=2^-10
  Constant : Constant  Value=10  OutDataTypeMode=uint8  OutDataType=fixdt(1, 16)  OutScaling=2^0  OutDataTypeStr=uint8
  Extract Bits : simulink/Logic and Bit Operations/Extract Bits  SystemSampleTime=-1  bitsToExtract=Range of bits  numBits=8  bitIdxRange=[4 5]  outScalingMode=Treat bit field as an integer
  Extract Bits1 : simulink/Logic and Bit Operations/Extract Bits  SystemSampleTime=-1  bitsToExtract=Range of bits  numBits=8  bitIdxRange=[0 3]  outScalingMode=Treat bit field as an integer
  Extract Bits2 : simulink/Logic and Bit Operations/Extract Bits  SystemSampleTime=-1  bitsToExtract=Range of bits  numBits=8  bitIdxRange=[5 5]  outScalingMode=Treat bit field as an integer
  Product : Product  OutDataType=fixdt(1, 16)  OutScaling=2^0  RndMeth=Zero
  Hour : Outport
  AM/PM : Outport  Port=2
  wires:
  Extract Bits2/1 -> AM/PM/1
  Extract Bits1/1 -> Add/2
  In1/1 -> Extract Bits2/1, Extract Bits1/1, Extract Bits/1
  Constant/1 -> Product/1
  Extract Bits/1 -> Product/2
  Product/1 -> Add/1
  Add/1 -> Hour/1

== system stm32f4_data_logger_ascii_rtc_demo/Date/Time/DS3231 Get Time/Convert/Convert Second/ Minute ==
  In1 : Inport
  Add : Sum  OutDataType=fixdt(1, 16)  OutScaling=2^-10
  Constant : Constant  Value=10  OutDataTypeMode=uint8  OutDataType=fixdt(1, 16)  OutScaling=2^0  OutDataTypeStr=uint8
  Extract Bits : simulink/Logic and Bit Operations/Extract Bits  SystemSampleTime=-1  bitsToExtract=Range of bits  numBits=8  bitIdxRange=[4 6]  outScalingMode=Treat bit field as an integer
  Extract Bits1 : simulink/Logic and Bit Operations/Extract Bits  SystemSampleTime=-1  bitsToExtract=Range of bits  numBits=8  bitIdxRange=[0 3]  outScalingMode=Treat bit field as an integer
  Product : Product  OutDataType=fixdt(1, 16)  OutScaling=2^0  RndMeth=Zero
  Out1 : Outport
  wires:
  Add/1 -> Out1/1
  Extract Bits1/1 -> Add/2
  Product/1 -> Add/1
  Extract Bits/1 -> Product/2
  Constant/1 -> Product/1
  In1/1 -> Extract Bits1/1, Extract Bits/1
